simulink model "boost_converter"  (R2021a)
settings: Solver=VariableStepAuto  StartTime=0.0  StopTime=1  RelTol=1e-3
libraries: spsSeriesRLCBranchLib x4, spsVoltageMeasurementLib x2, spsCurrentMeasurementLib x2, spsDCVoltageSourceLib x1, spsDiodeLib x1, spsIdealSwitchLib x1, eePwmGenerator x1, spspowerguiLib x1
settings Model: Creator=ASUS  LastModifiedBy=ASUS

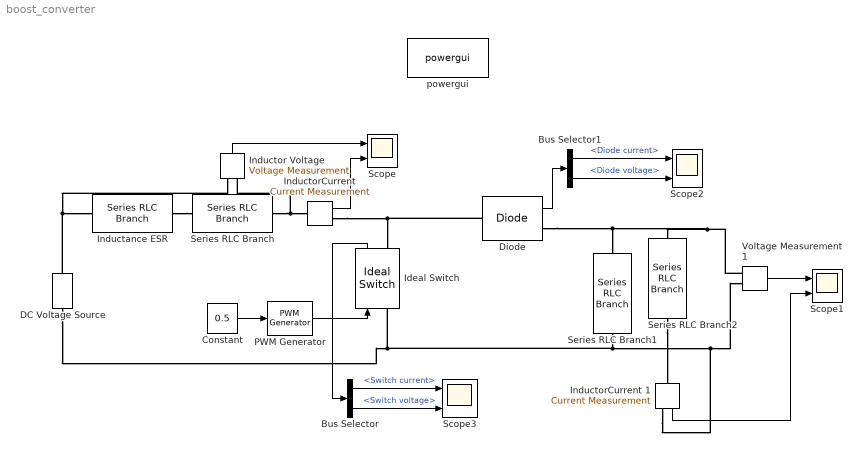
== system boost_converter ==
  Bus Selector : BusSelector  OutputSignals=Switch current,Switch voltage
  Bus Selector1 : BusSelector  OutputSignals=Diode current,Diode voltage
  Constant : Constant  Value=0.5
  DC Voltage Source : spsDCVoltageSourceLib/DC Voltage Source  Amplitude=15  Measurements=None
  Diode : spsDiodeLib/Diode  Ron=0.000000001  Lon=0  Vf=0.001  IC=0  UseSnubber=0  Rs=500  Cs=250e-6  Measurements=on
  Ideal Switch : spsIdealSwitchLib/Ideal Switch  Ron=0.001  Lon=0  IC=0  Rs=1e5  Cs=inf  Measurements=on
  Inductance ESR : spsSeriesRLCBranchLib/Series RLC Branch  LConnTagsString=__new0  RConnTagsString=__new0  BranchType=R  Resistance=57e-3  Inductance=1e-3  SetiL0=off  InitialCurrent=0  Capacitance=1e-6  Setx0=off  InitialVoltage=0  Measurements=None
  Inductor Voltage : spsVoltageMeasurementLib/Voltage Measurement  PhasorSimulation=off  OutputType=Complex  PSBequivalent=0
  "InductorCurrent " : spsCurrentMeasurementLib/Current Measurement  PhasorSimulation=off  OutputType=Complex  PSBequivalent=0
  InductorCurrent 1 : spsCurrentMeasurementLib/Current Measurement  PhasorSimulation=off  OutputType=Complex  PSBequivalent=0
  PWM Generator : eePwmGenerator/PWM Generator  CarrCount=Up  Tper=2e-6  Ts=2e-7
  Scope{,1..3} (4 alike) : Scope  NumInputPorts=2
  Series RLC Branch : spsSeriesRLCBranchLib/Series RLC Branch  LConnTagsString=__new0  RConnTagsString=__new0  BranchType=L  Resistance=1  Inductance=7.2e-6  SetiL0=off  InitialCurrent=0  Capacitance=1e-6  Setx0=off  InitialVoltage=0  Measurements=None
  Series RLC Branch1 : spsSeriesRLCBranchLib/Series RLC Branch  LConnTagsString=__new0  RConnTagsString=__new0  BranchType=C  Resistance=1  Inductance=1e-3  SetiL0=off  InitialCurrent=0  Capacitance=4.86e-6  Setx0=off  InitialVoltage=0  Measurements=None
  Series RLC Branch2 : spsSeriesRLCBranchLib/Series RLC Branch  LConnTagsString=__new0  RConnTagsString=__new0  BranchType=R  Resistance=57.6  Inductance=1e-3  SetiL0=off  InitialCurrent=0  Capacitance=1e-6  Setx0=off  InitialVoltage=0  Measurements=None
  Voltage Measurement1 : spsVoltageMeasurementLib/Voltage Measurement  PhasorSimulation=off  OutputType=Complex  PSBequivalent=0
  powergui : spspowerguiLib/powergui  Priority=1  SimulationMode=Continuous  SampleTime=50e-6  frequency=60  Iterations=50  frequencyindice=0  Pbase=100e6  ErrMax=1e-4  UnitsV=kV  UnitsW=MW  buscounter=0  FunctionMessages=off  echomessages=off  EnableUseOfTLC=off  CurrentSourceSwitches=off  DisableSnubberDevices=off  DisableRonSwitches=off  DisableVfSwitches=off  DisplayEquations=off  AutomaticDiscreteSolvers=off  SolverType=Tustin/Backward Euler (TBE)  Interpol=off  ExternalGateDelay=off  methode=off  Ts=100  x0status=blocks  SPID=on  SwTol=0  HookPort=off  NonlinearTolerance=1e-4  nMaxIteration=100  ContinueOnMaxIteration=off  RestoreLinks=warning  ResistiveCurrentMeasurement=off  Frange=[0:2:500]  Ylog=off  Xlog=on  ShowGrid=off  save=off  variable=ZData  structure=0  ZoomFFT=off  StartTime=0.0  cycles=1  DisplayStyle=1  fundamental=60  FreqAxis=off  MaxFrequency=1000  frequencyindicesteady=1  RmsSteady=1  display=off
  wires:
  Inductor Voltage/1 -> Scope/1
  "InductorCurrent "/1 -> Scope/2
  Ideal Switch/1 -> Bus Selector/1
  Bus Selector/1 -> Scope3/1  "<Switch current>"
  Bus Selector/2 -> Scope3/2  "<Switch voltage>"
  Voltage Measurement1/1 -> Scope1/1
  Bus Selector1/1 -> Scope2/1  "<Diode current>"
  Bus Selector1/2 -> Scope2/2  "<Diode voltage>"
  Diode/1 -> Bus Selector1/1
  Constant/1 -> PWM Generator/1
  PWM Generator/1 -> Ideal Switch/1
  InductorCurrent 1/1 -> Scope1/2
  connections:
  DC Voltage Source/RConn1 -- Inductor Voltage/LConn1 -- Inductance ESR/LConn1
  Diode/LConn1 -- "InductorCurrent "/RConn1 -- Ideal Switch/RConn1
  DC Voltage Source/LConn1 -- Ideal Switch/LConn1 -- Voltage Measurement1/LConn2 -- InductorCurrent 1/RConn1 -- Series RLC Branch1/RConn1
  Diode/RConn1 -- Voltage Measurement1/LConn1 -- Series RLC Branch2/LConn1 -- Series RLC Branch1/LConn1
  Series RLC Branch/RConn1 -- Inductor Voltage/LConn2 -- "InductorCurrent "/LConn1
  Series RLC Branch2/RConn1 -- InductorCurrent 1/LConn1
  Inductance ESR/RConn1 -- Series RLC Branch/LConn1
